simulink model "TimeDelay_DiffParameters"  (R2019b)
settings: Solver=VariableStepAuto  StartTime=0.0  StopTime=1500  RelTol=1e-3
values from neighbouring files (symbols this model uses):
  tau1 = 15    [SmithControl.m]    (also in TimeDelayParameters.m; positivity_matrix.m)
  tau2 = 20    [SmithControl.m]    (also in TimeDelayParameters.m = 30; positivity_matrix.m = 30)
  th1 = 0.85    [AP_TimeDelay.m]    (also in SmithControl.m; TimeDelayParameters.m = 0.32; positivity_matrix.m; rscale.m)
  th2 = 50    [AP_TimeDelay.m]    (also in SmithControl.m; TimeDelayParameters.m; positivity_matrix.m; rscale.m)
  th3 = 60    [AP_TimeDelay.m]    (also in SmithControl.m; TimeDelayParameters.m = 70; positivity_matrix.m; rscale.m)
  th4 = 5    [AP_TimeDelay.m]    (also in SmithControl.m; TimeDelayParameters.m = 2.7; positivity_matrix.m; rscale.m)
  th5 = 20    [AP_TimeDelay.m]    (also in SmithControl.m; TimeDelayParameters.m = 22; positivity_matrix.m; rscale.m)
settings Model: Creator=akshita_jain  LastModifiedBy=akshita_jain

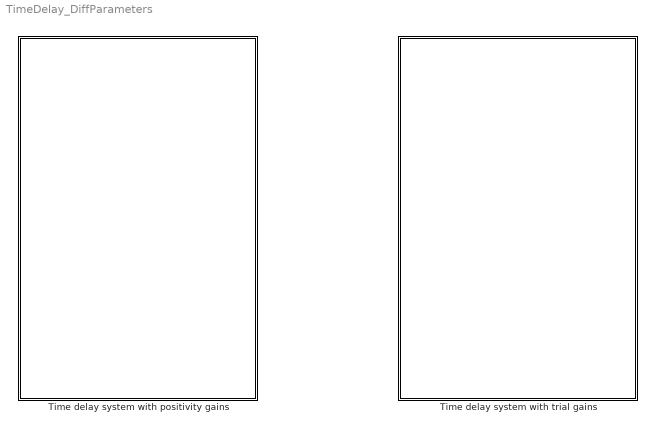
== system TimeDelay_DiffParameters ==
  Time delay system with positivity gains : Subsystem
  Time delay system with trial gains : Subsystem

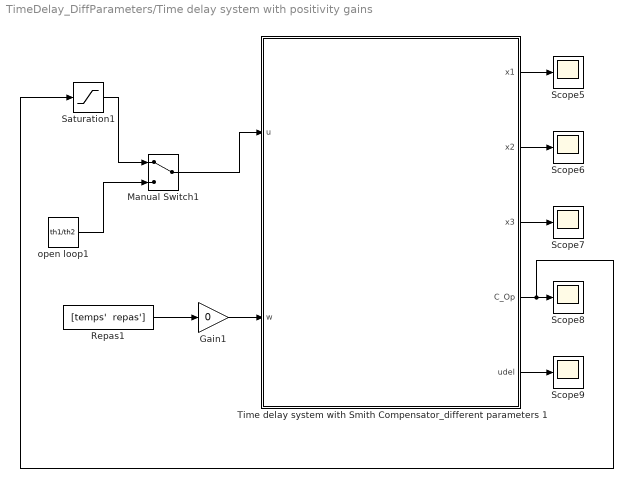
== system TimeDelay_DiffParameters/Time delay system with positivity gains ==
  Gain1 : Gain  Gain=0
  Manual Switch1 : ManualSwitch
  Repas1 : FromWorkspace  VariableName="[temps'  repas']"  SampleTime=0
  Saturation1 : Saturate  UpperLimit=2  LowerLimit=0
  Scope{5..9} (5 alike) : Scope
  Time delay system with Smith Compensator_different parameters 1 : Subsystem
  open loop1 : Constant  Value=th1/th2
  wires:
  Manual Switch1/1 -> Time delay system with Smith Compensator_different parameters 1/1(u)
  Gain1/1 -> Time delay system with Smith Compensator_different parameters 1/2(w)
  Time delay system with Smith Compensator_different parameters 1/3(x3) -> Scope7/1
  Time delay system with Smith Compensator_different parameters 1/2(x2) -> Scope6/1
  Time delay system with Smith Compensator_different parameters 1/5(udel) -> Scope9/1
  Saturation1/1 -> Manual Switch1/1
  Time delay system with Smith Compensator_different parameters 1/1(x1) -> Scope5/1
  Time delay system with Smith Compensator_different parameters 1/4(C_Op) -> Saturation1/1, Scope8/1
  Repas1/1 -> Gain1/1
  open loop1/1 -> Manual Switch1/2

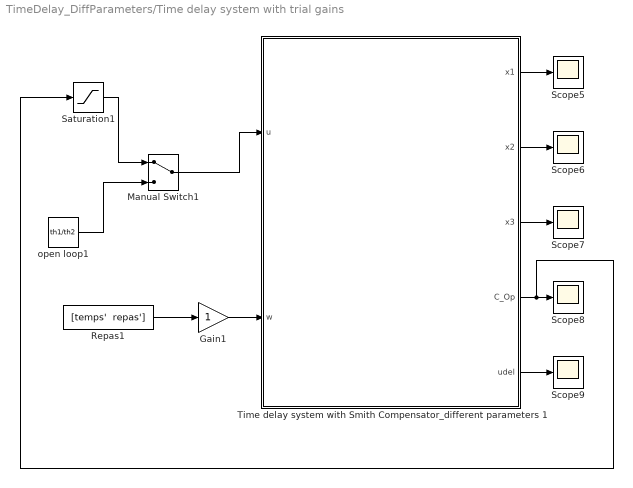
== system TimeDelay_DiffParameters/Time delay system with trial gains ==
  Gain1 : Gain
  Manual Switch1 : ManualSwitch
  Repas1 : FromWorkspace  VariableName="[temps'  repas']"  SampleTime=0
  Saturation1 : Saturate  UpperLimit=2  LowerLimit=0
  Scope{5..9} (5 alike) : Scope
  Time delay system with Smith Compensator_different parameters 1 : Subsystem
  open loop1 : Constant  Value=th1/th2
  wires:
  Manual Switch1/1 -> Time delay system with Smith Compensator_different parameters 1/1(u)
  Gain1/1 -> Time delay system with Smith Compensator_different parameters 1/2(w)
  Time delay system with Smith Compensator_different parameters 1/3(x3) -> Scope7/1
  Time delay system with Smith Compensator_different parameters 1/2(x2) -> Scope6/1
  Time delay system with Smith Compensator_different parameters 1/5(udel) -> Scope9/1
  Saturation1/1 -> Manual Switch1/1
  Time delay system with Smith Compensator_different parameters 1/1(x1) -> Scope5/1
  Time delay system with Smith Compensator_different parameters 1/4(C_Op) -> Saturation1/1, Scope8/1
  Repas1/1 -> Gain1/1
  open loop1/1 -> Manual Switch1/2

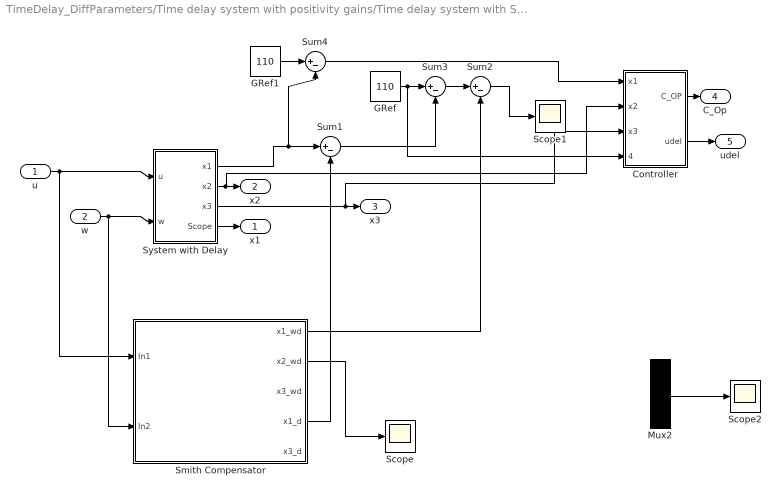
== system TimeDelay_DiffParameters/Time delay system with positivity gains/Time delay system with Smith Compensator_different parameters 1 ==
  u : Inport
  w : Inport  Port=2
  "Controller " : Subsystem
  GRef : Constant  Value=110
  GRef1 : Constant  Value=110
  Mux2 : Mux
  Scope : Scope
  Scope1 : Scope
  Scope2 : Scope
  Smith Compensator : Subsystem
  Sum{1..4} (4 alike) : Sum  Inputs=|+-
  System with Delay : Subsystem
  x1 : Outport
  x2 : Outport  Port=2
  x3 : Outport  Port=3
  C_Op : Outport  Port=4
  udel : Outport  Port=5
  wires:
  u/1 -> Smith Compensator/1(In1), System with Delay/1(u)
  w/1 -> Smith Compensator/2(In2), System with Delay/2(w)
  System with Delay/4(Scope) -> x1/1
  System with Delay/1(x1) -> Sum1/1, Sum4/2
  Smith Compensator/4(x1_d) -> Sum1/2
  Smith Compensator/1(x1_wd) -> Sum2/2
  Sum2/1 -> Scope1/1
  GRef/1 -> "Controller "/4(x1_ref), Sum3/1
  System with Delay/2(x2) -> "Controller "/2(x2), x2/1
  System with Delay/3(x3) -> "Controller "/3(x3), x3/1
  "Controller "/1(C_OP) -> C_Op/1
  "Controller "/2(udel) -> udel/1
  Mux2/1 -> Scope2/1
  Smith Compensator/2(x2_wd) -> Scope/1
  Sum3/1 -> Sum2/1
  GRef1/1 -> Sum4/1
  Sum1/1 -> Sum3/2
  Sum4/1 -> "Controller "/1(x1)

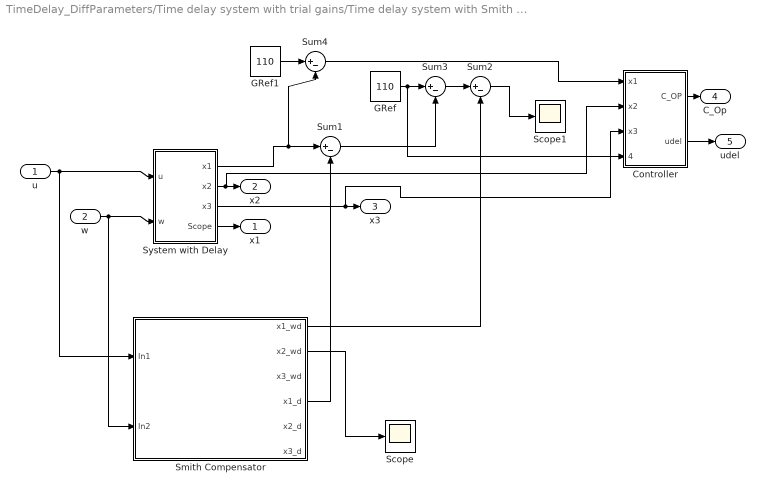
== system TimeDelay_DiffParameters/Time delay system with trial gains/Time delay system with Smith Compensator_different parameters 1 ==
  u : Inport
  w : Inport  Port=2
  "Controller " : Subsystem
  GRef : Constant  Value=110
  GRef1 : Constant  Value=110
  Scope : Scope
  Scope1 : Scope
  Smith Compensator : Subsystem
  Sum{1..4} (4 alike) : Sum  Inputs=|+-
  System with Delay : Subsystem
  x1 : Outport
  x2 : Outport  Port=2
  x3 : Outport  Port=3
  C_Op : Outport  Port=4
  udel : Outport  Port=5
  wires:
  u/1 -> Smith Compensator/1(In1), System with Delay/1(u)
  w/1 -> Smith Compensator/2(In2), System with Delay/2(w)
  System with Delay/4(Scope) -> x1/1
  System with Delay/1(x1) -> Sum1/1, Sum4/2
  Smith Compensator/4(x1_d) -> Sum1/2
  Smith Compensator/1(x1_wd) -> Sum2/2
  Sum2/1 -> Scope1/1
  GRef/1 -> "Controller "/4(x1_ref), Sum3/1
  System with Delay/2(x2) -> "Controller "/2(x2), x2/1
  System with Delay/3(x3) -> "Controller "/3(x3), x3/1
  "Controller "/1(C_OP) -> C_Op/1
  "Controller "/2(udel) -> udel/1
  Smith Compensator/2(x2_wd) -> Scope/1
  Sum3/1 -> Sum2/1
  GRef1/1 -> Sum4/1
  Sum1/1 -> Sum3/2
  Sum4/1 -> "Controller "/1(x1)

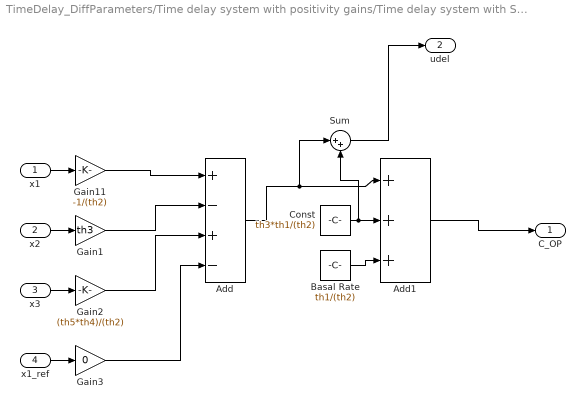
== system TimeDelay_DiffParameters/Time delay system with positivity gains/Time delay system with Smith Compensator_different parameters 1/Controller  ==
  x1 : Inport
  x2 : Inport  Port=2
  x3 : Inport  Port=3
  x1_ref : Inport  Port=4
  Add : Sum  Inputs=+-+-
  Add1 : Sum  Inputs=+++
  Basal Rate : Constant  Value=th1/(th2)  VectorParams1D=off
  Const : Constant  Value=th3*th1/(th2)  VectorParams1D=off
  Gain1 : Gain  Gain=th3
  Gain11 : Gain  Gain=-1/(th2)
  Gain2 : Gain  Gain=(th5*th4)/(th2)
  Gain3 : Gain  Gain=0
  Sum : Sum  Inputs=|++
  C_OP : Outport
  udel : Outport  Port=2
  wires:
  x1/1 -> Gain11/1
  x2/1 -> Gain1/1
  x3/1 -> Gain2/1
  Gain11/1 -> Add/1
  Gain1/1 -> Add/2
  Gain2/1 -> Add/3
  Add/1 -> Sum/1, Add1/1
  Const/1 -> Add1/2, Sum/2
  Basal Rate/1 -> Add1/3
  Add1/1 -> C_OP/1
  Sum/1 -> udel/1
  x1_ref/1 -> Gain3/1
  Gain3/1 -> Add/4

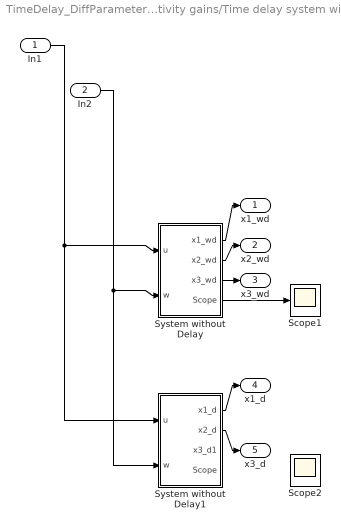
== system TimeDelay_DiffParameters/Time delay system with positivity gains/Time delay system with Smith Compensator_different parameters 1/Smith Compensator ==
  In1 : Inport
  In2 : Inport  Port=2
  Scope1 : Scope
  Scope2 : Scope
  System without Delay : Subsystem
  System without Delay1 : Subsystem
  x1_wd : Outport
  x2_wd : Outport  Port=2
  x3_wd : Outport  Port=3
  x1_d : Outport  Port=4
  x3_d : Outport  Port=5
  wires:
  System without Delay/3(x3_wd) -> x3_wd/1
  System without Delay/2(x2_wd) -> x2_wd/1
  System without Delay/4(Scope) -> Scope1/1
  System without Delay1/1(x1_d) -> x1_d/1
  System without Delay/1(x1_wd) -> x1_wd/1
  System without Delay1/2(x2_d) -> x3_d/1
  In2/1 -> System without Delay1/2(w), System without Delay/2(w)
  In1/1 -> System without Delay1/1(u), System without Delay/1(u)

== system TimeDelay_DiffParameters/Time delay system with positivity gains/Time delay system with Smith Compensator_different parameters 1/System with Delay ==
  u : Inport
  w : Inport  Port=2
  CHO : Subsystem
  Glucose : Subsystem
  Insulin Plasma : Subsystem
  x1 : Outport
  x2 : Outport  Port=2
  x3 : Outport  Port=3
  Scope : Outport  Port=4
  wires:
  Glucose/1(Out1) -> Scope/1
  Glucose/2(x1) -> x1/1
  w/1 -> CHO/1(w)
  Insulin Plasma/1(x2) -> x2/1, Glucose/1(x2)
  u/1 -> Insulin Plasma/1(u)
  CHO/1(x3) -> x3/1, Glucose/2(x3)

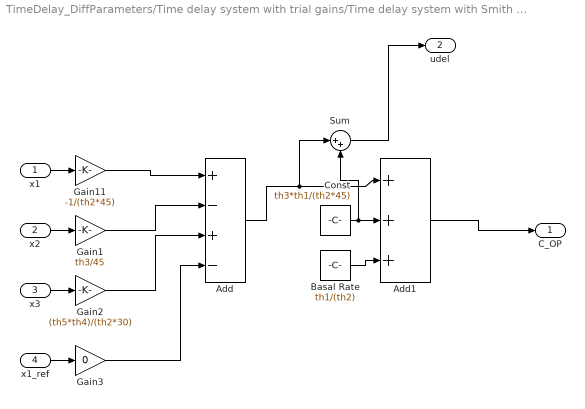
== system TimeDelay_DiffParameters/Time delay system with trial gains/Time delay system with Smith Compensator_different parameters 1/Controller  ==
  x1 : Inport
  x2 : Inport  Port=2
  x3 : Inport  Port=3
  x1_ref : Inport  Port=4
  Add : Sum  Inputs=+-+-
  Add1 : Sum  Inputs=+++
  Basal Rate : Constant  Value=th1/(th2)  VectorParams1D=off
  Const : Constant  Value=th3*th1/(th2*45)  VectorParams1D=off
  Gain1 : Gain  Gain=th3/45
  Gain11 : Gain  Gain=-1/(th2*45)
  Gain2 : Gain  Gain=(th5*th4)/(th2*30)
  Gain3 : Gain  Gain=0
  Sum : Sum  Inputs=|++
  C_OP : Outport
  udel : Outport  Port=2
  wires:
  x1/1 -> Gain11/1
  x2/1 -> Gain1/1
  x3/1 -> Gain2/1
  Gain11/1 -> Add/1
  Gain1/1 -> Add/2
  Gain2/1 -> Add/3
  Add/1 -> Sum/1, Add1/1
  Const/1 -> Add1/2, Sum/2
  Basal Rate/1 -> Add1/3
  Add1/1 -> C_OP/1
  Sum/1 -> udel/1
  x1_ref/1 -> Gain3/1
  Gain3/1 -> Add/4

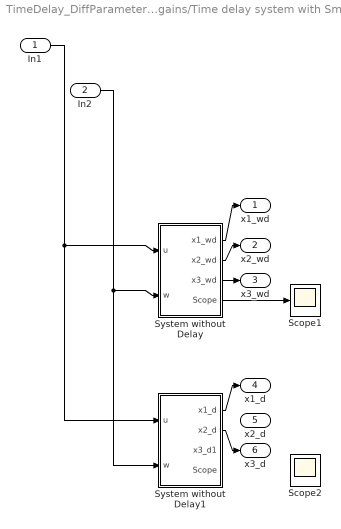
== system TimeDelay_DiffParameters/Time delay system with trial gains/Time delay system with Smith Compensator_different parameters 1/Smith Compensator ==
  In1 : Inport
  In2 : Inport  Port=2
  Scope1 : Scope
  Scope2 : Scope
  System without Delay : Subsystem
  System without Delay1 : Subsystem
  x1_wd : Outport
  x2_wd : Outport  Port=2
  x3_wd : Outport  Port=3
  x1_d : Outport  Port=4
  x2_d : Outport  Port=5
  x3_d : Outport  Port=6
  wires:
  System without Delay/3(x3_wd) -> x3_wd/1
  System without Delay/2(x2_wd) -> x2_wd/1
  System without Delay/4(Scope) -> Scope1/1
  System without Delay1/1(x1_d) -> x1_d/1
  System without Delay/1(x1_wd) -> x1_wd/1
  System without Delay1/2(x2_d) -> x3_d/1
  In2/1 -> System without Delay1/2(w), System without Delay/2(w)
  In1/1 -> System without Delay1/1(u), System without Delay/1(u)

== system TimeDelay_DiffParameters/Time delay system with trial gains/Time delay system with Smith Compensator_different parameters 1/System with Delay ==
  u : Inport
  w : Inport  Port=2
  CHO : Subsystem
  Glucose : Subsystem
  Insulin Plasma : Subsystem
  Scope1 : Scope
  x1 : Outport
  x2 : Outport  Port=2
  x3 : Outport  Port=3
  Scope : Outport  Port=4
  wires:
  Glucose/1(Out1) -> Scope/1
  Glucose/2(x1) -> x1/1
  w/1 -> CHO/1(w)
  Insulin Plasma/1(x2) -> Scope1/1, x2/1, Glucose/1(x2)
  CHO/1(x3) -> x3/1, Glucose/2(x3)
  u/1 -> Insulin Plasma/1(u)

== system TimeDelay_DiffParameters/Time delay system with positivity gains/Time delay system with Smith Compensator_different parameters 1/Smith Compensator/System without Delay ==
  u : Inport
  w : Inport  Port=2
  CHO : Subsystem
  Glucose : Subsystem
  Insulin Plasma : Subsystem
  x1_wd : Outport
  x2_wd : Outport  Port=2
  x3_wd : Outport  Port=3
  Scope : Outport  Port=4
  wires:
  Glucose/2(x1) -> x1_wd/1
  w/1 -> CHO/1(In2)
  Insulin Plasma/1(x2) -> x2_wd/1, Glucose/1(In1)
  u/1 -> Insulin Plasma/1(In1)
  CHO/1(x3) -> x3_wd/1, Glucose/2(In2)
  Glucose/1(Out1) -> Scope/1

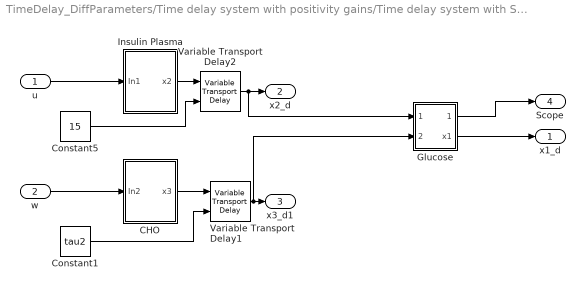
== system TimeDelay_DiffParameters/Time delay system with positivity gains/Time delay system with Smith Compensator_different parameters 1/Smith Compensator/System without Delay1 ==
  u : Inport
  w : Inport  Port=2
  CHO : Subsystem
  Constant1 : Constant  Value=tau2
  Constant5 : Constant  Value=15
  Glucose : Subsystem
  Insulin Plasma : Subsystem
  Variable Transport Delay1 : VariableTransportDelay  VariableDelayType=Variable transport delay  MaximumDelay=30
  Variable Transport Delay2 : VariableTransportDelay  VariableDelayType=Variable transport delay  MaximumDelay=20  InitialOutput=0.0167
  x1_d : Outport
  x2_d : Outport  Port=2
  x3_d1 : Outport  Port=3
  Scope : Outport  Port=4
  wires:
  Glucose/2(x1) -> x1_d/1
  w/1 -> CHO/1(In2)
  u/1 -> Insulin Plasma/1(In1)
  Variable Transport Delay2/1 -> x2_d/1, Glucose/1(In1)
  Insulin Plasma/1(x2) -> Variable Transport Delay2/1
  Constant5/1 -> Variable Transport Delay2/2
  CHO/1(x3) -> Variable Transport Delay1/1
  Variable Transport Delay1/1 -> x3_d1/1, Glucose/2(In2)
  Constant1/1 -> Variable Transport Delay1/2
  Glucose/1(Out1) -> Scope/1

== system TimeDelay_DiffParameters/Time delay system with positivity gains/Time delay system with Smith Compensator_different parameters 1/System with Delay/CHO ==
  w : Inport
  Add6 : Sum  Inputs=-+
  Constant6 : Constant  Value=30  VectorParams1D=off
  Gain12 : Gain  Gain=1/th5
  Gain13 : Gain  Gain=1/th5
  Integrator6 : Integrator  ZeroCross=off
  Variable Transport Delay3 : VariableTransportDelay  VariableDelayType=Variable transport delay  MaximumDelay=30
  x3 : Outport
  wires:
  Variable Transport Delay3/1 -> Gain12/1
  w/1 -> Variable Transport Delay3/1
  Integrator6/1 -> x3/1, Gain13/1
  Add6/1 -> Integrator6/1
  Constant6/1 -> Variable Transport Delay3/2
  Gain13/1 -> Add6/1
  Gain12/1 -> Add6/2

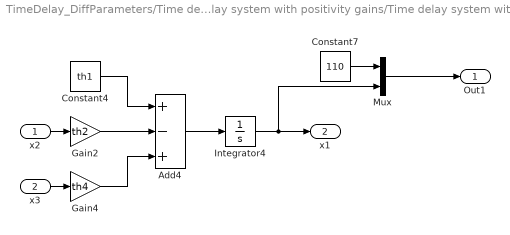
== system TimeDelay_DiffParameters/Time delay system with positivity gains/Time delay system with Smith Compensator_different parameters 1/System with Delay/Glucose ==
  x2 : Inport
  x3 : Inport  Port=2
  Add4 : Sum  Inputs=+-+
  Constant4 : Constant  Value=th1  VectorParams1D=off
  Constant7 : Constant  Value=110  VectorParams1D=off
  Gain2 : Gain  Gain=th2
  Gain4 : Gain  Gain=th4
  Integrator4 : Integrator  InitialCondition=110  ZeroCross=off
  Mux : Mux  Inputs=2
  Out1 : Outport
  x1 : Outport  Port=2
  wires:
  Gain2/1 -> Add4/2
  x3/1 -> Gain4/1
  x2/1 -> Gain2/1
  Mux/1 -> Out1/1
  Add4/1 -> Integrator4/1
  Constant4/1 -> Add4/1
  Integrator4/1 -> x1/1, Mux/2
  Gain4/1 -> Add4/3
  Constant7/1 -> Mux/1

== system TimeDelay_DiffParameters/Time delay system with positivity gains/Time delay system with Smith Compensator_different parameters 1/System with Delay/Insulin Plasma ==
  u : Inport
  Add5 : Sum  Inputs=-+
  Constant5 : Constant  Value=tau1
  Gain10 : Gain  Gain=1/th3
  Gain11 : Gain  Gain=1/th3
  Integrator5 : Integrator  InitialCondition=th1/(th2)  ZeroCross=off
  Variable Transport Delay2 : VariableTransportDelay  VariableDelayType=Variable transport delay  MaximumDelay=20
  x2 : Outport
  wires:
  Add5/1 -> Integrator5/1
  Gain11/1 -> Add5/1
  Gain10/1 -> Add5/2
  Constant5/1 -> Variable Transport Delay2/2
  Integrator5/1 -> x2/1, Gain11/1
  u/1 -> Variable Transport Delay2/1
  Variable Transport Delay2/1 -> Gain10/1

== system TimeDelay_DiffParameters/Time delay system with trial gains/Time delay system with Smith Compensator_different parameters 1/Smith Compensator/System without Delay ==
  u : Inport
  w : Inport  Port=2
  CHO : Subsystem
  Glucose : Subsystem
  Insulin Plasma : Subsystem
  x1_wd : Outport
  x2_wd : Outport  Port=2
  x3_wd : Outport  Port=3
  Scope : Outport  Port=4
  wires:
  Glucose/2(x1) -> x1_wd/1
  w/1 -> CHO/1(In2)
  Insulin Plasma/1(x2) -> x2_wd/1, Glucose/1(In1)
  u/1 -> Insulin Plasma/1(In1)
  CHO/1(x3) -> x3_wd/1, Glucose/2(In2)
  Glucose/1(Out1) -> Scope/1

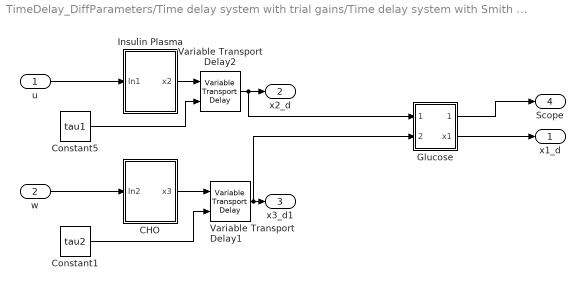
== system TimeDelay_DiffParameters/Time delay system with trial gains/Time delay system with Smith Compensator_different parameters 1/Smith Compensator/System without Delay1 ==
  u : Inport
  w : Inport  Port=2
  CHO : Subsystem
  Constant1 : Constant  Value=tau2
  Constant5 : Constant  Value=tau1
  Glucose : Subsystem
  Insulin Plasma : Subsystem
  Variable Transport Delay1 : VariableTransportDelay  VariableDelayType=Variable transport delay  MaximumDelay=30
  Variable Transport Delay2 : VariableTransportDelay  VariableDelayType=Variable transport delay  MaximumDelay=20
  x1_d : Outport
  x2_d : Outport  Port=2
  x3_d1 : Outport  Port=3
  Scope : Outport  Port=4
  wires:
  Glucose/2(x1) -> x1_d/1
  w/1 -> CHO/1(In2)
  u/1 -> Insulin Plasma/1(In1)
  Variable Transport Delay2/1 -> x2_d/1, Glucose/1(In1)
  Insulin Plasma/1(x2) -> Variable Transport Delay2/1
  Constant5/1 -> Variable Transport Delay2/2
  CHO/1(x3) -> Variable Transport Delay1/1
  Variable Transport Delay1/1 -> x3_d1/1, Glucose/2(In2)
  Constant1/1 -> Variable Transport Delay1/2
  Glucose/1(Out1) -> Scope/1

== system TimeDelay_DiffParameters/Time delay system with trial gains/Time delay system with Smith Compensator_different parameters 1/System with Delay/CHO ==
  w : Inport
  Add6 : Sum  Inputs=-+
  Constant6 : Constant  Value=30  VectorParams1D=off
  Gain12 : Gain  Gain=1/th5
  Gain13 : Gain  Gain=1/th5
  Integrator6 : Integrator  ZeroCross=off
  Variable Transport Delay3 : VariableTransportDelay  VariableDelayType=Variable transport delay  MaximumDelay=30
  x3 : Outport
  wires:
  Variable Transport Delay3/1 -> Gain12/1
  w/1 -> Variable Transport Delay3/1
  Integrator6/1 -> x3/1, Gain13/1
  Add6/1 -> Integrator6/1
  Constant6/1 -> Variable Transport Delay3/2
  Gain13/1 -> Add6/1
  Gain12/1 -> Add6/2

== system TimeDelay_DiffParameters/Time delay system with trial gains/Time delay system with Smith Compensator_different parameters 1/System with Delay/Glucose ==
  x2 : Inport
  x3 : Inport  Port=2
  Add4 : Sum  Inputs=+-+
  Constant4 : Constant  Value=th1  VectorParams1D=off
  Constant7 : Constant  Value=110  VectorParams1D=off
  Gain2 : Gain  Gain=th2
  Gain4 : Gain  Gain=th4
  Integrator4 : Integrator  InitialCondition=110  ZeroCross=off
  Mux : Mux  Inputs=2
  Out1 : Outport
  x1 : Outport  Port=2
  wires:
  Gain2/1 -> Add4/2
  x3/1 -> Gain4/1
  x2/1 -> Gain2/1
  Mux/1 -> Out1/1
  Add4/1 -> Integrator4/1
  Constant4/1 -> Add4/1
  Integrator4/1 -> x1/1, Mux/2
  Gain4/1 -> Add4/3
  Constant7/1 -> Mux/1

== system TimeDelay_DiffParameters/Time delay system with trial gains/Time delay system with Smith Compensator_different parameters 1/System with Delay/Insulin Plasma ==
  u : Inport
  Add5 : Sum  Inputs=-+
  Constant5 : Constant  Value=tau1
  Gain10 : Gain  Gain=th1/th2*th3
  Gain11 : Gain  Gain=1/th3
  Integrator5 : Integrator  InitialCondition=th1/(th2)  ZeroCross=off
  Variable Transport Delay2 : VariableTransportDelay  VariableDelayType=Variable transport delay  MaximumDelay=20  InitialOutput=th1/th2
  x2 : Outport
  wires:
  Gain11/1 -> Add5/1
  Gain10/1 -> Add5/2
  Constant5/1 -> Variable Transport Delay2/2
  u/1 -> Variable Transport Delay2/1
  Variable Transport Delay2/1 -> Gain10/1
  Integrator5/1 -> x2/1, Gain11/1
  Add5/1 -> Integrator5/1

== system TimeDelay_DiffParameters/Time delay system with positivity gains/Time delay system with Smith Compensator_different parameters 1/Smith Compensator/System without Delay/CHO ==
  In2 : Inport
  Add6 : Sum  Inputs=-+
  Gain12 : Gain  Gain=1/th5
  Gain13 : Gain  Gain=1/th5
  Integrator6 : Integrator  ZeroCross=off
  x3 : Outport
  wires:
  In2/1 -> Gain12/1
  Integrator6/1 -> x3/1, Gain13/1
  Add6/1 -> Integrator6/1
  Gain13/1 -> Add6/1
  Gain12/1 -> Add6/2

== system TimeDelay_DiffParameters/Time delay system with positivity gains/Time delay system with Smith Compensator_different parameters 1/Smith Compensator/System without Delay/Glucose ==
  In1 : Inport
  In2 : Inport  Port=2
  Add4 : Sum  Inputs=+-+
  Constant4 : Constant  Value=th1  VectorParams1D=off
  Constant7 : Constant  Value=110  VectorParams1D=off
  Gain2 : Gain  Gain=th2
  Gain4 : Gain  Gain=th4
  Integrator4 : Integrator  InitialCondition=110  ZeroCross=off
  Mux : Mux  Inputs=2
  Out1 : Outport
  x1 : Outport  Port=2
  wires:
  Gain2/1 -> Add4/2
  In2/1 -> Gain4/1
  In1/1 -> Gain2/1
  Mux/1 -> Out1/1
  Add4/1 -> Integrator4/1
  Constant4/1 -> Add4/1
  Integrator4/1 -> x1/1, Mux/2
  Gain4/1 -> Add4/3
  Constant7/1 -> Mux/1

== system TimeDelay_DiffParameters/Time delay system with positivity gains/Time delay system with Smith Compensator_different parameters 1/Smith Compensator/System without Delay/Insulin Plasma ==
  In1 : Inport
  Add5 : Sum  Inputs=-+
  Gain10 : Gain  Gain=1/th3
  Gain11 : Gain  Gain=1/th3
  Integrator5 : Integrator  InitialCondition=0.017  ZeroCross=off
  x2 : Outport
  wires:
  Add5/1 -> Integrator5/1
  Gain11/1 -> Add5/1
  In1/1 -> Gain10/1
  Gain10/1 -> Add5/2
  Integrator5/1 -> x2/1, Gain11/1

== system TimeDelay_DiffParameters/Time delay system with positivity gains/Time delay system with Smith Compensator_different parameters 1/Smith Compensator/System without Delay1/CHO ==
  In2 : Inport
  Add6 : Sum  Inputs=-+
  Gain12 : Gain  Gain=1/th5
  Gain13 : Gain  Gain=1/th5
  Integrator6 : Integrator  ZeroCross=off
  x3 : Outport
  wires:
  In2/1 -> Gain12/1
  Integrator6/1 -> x3/1, Gain13/1
  Add6/1 -> Integrator6/1
  Gain13/1 -> Add6/1
  Gain12/1 -> Add6/2

== system TimeDelay_DiffParameters/Time delay system with positivity gains/Time delay system with Smith Compensator_different parameters 1/Smith Compensator/System without Delay1/Glucose ==
  In1 : Inport
  In2 : Inport  Port=2
  Add4 : Sum  Inputs=+-+
  Constant4 : Constant  Value=th1  VectorParams1D=off
  Constant7 : Constant  Value=110  VectorParams1D=off
  Gain2 : Gain  Gain=th2
  Gain4 : Gain  Gain=th4
  Integrator4 : Integrator  InitialCondition=110  ZeroCross=off
  Mux : Mux  Inputs=2
  Out1 : Outport
  x1 : Outport  Port=2
  wires:
  Gain2/1 -> Add4/2
  In2/1 -> Gain4/1
  In1/1 -> Gain2/1
  Mux/1 -> Out1/1
  Add4/1 -> Integrator4/1
  Constant4/1 -> Add4/1
  Integrator4/1 -> x1/1, Mux/2
  Gain4/1 -> Add4/3
  Constant7/1 -> Mux/1

== system TimeDelay_DiffParameters/Time delay system with positivity gains/Time delay system with Smith Compensator_different parameters 1/Smith Compensator/System without Delay1/Insulin Plasma ==
  In1 : Inport
  Add5 : Sum  Inputs=-+
  Gain10 : Gain  Gain=1/th3
  Gain11 : Gain  Gain=1/th3
  Integrator5 : Integrator  InitialCondition=0.017  ZeroCross=off
  x2 : Outport
  wires:
  Add5/1 -> Integrator5/1
  Gain11/1 -> Add5/1
  In1/1 -> Gain10/1
  Gain10/1 -> Add5/2
  Integrator5/1 -> x2/1, Gain11/1

== system TimeDelay_DiffParameters/Time delay system with trial gains/Time delay system with Smith Compensator_different parameters 1/Smith Compensator/System without Delay/CHO ==
  In2 : Inport
  Add6 : Sum  Inputs=-+
  Gain12 : Gain  Gain=1/th5
  Gain13 : Gain  Gain=1/th5
  Integrator6 : Integrator  ZeroCross=off
  x3 : Outport
  wires:
  In2/1 -> Gain12/1
  Integrator6/1 -> x3/1, Gain13/1
  Add6/1 -> Integrator6/1
  Gain13/1 -> Add6/1
  Gain12/1 -> Add6/2

== system TimeDelay_DiffParameters/Time delay system with trial gains/Time delay system with Smith Compensator_different parameters 1/Smith Compensator/System without Delay/Glucose ==
  In1 : Inport
  In2 : Inport  Port=2
  Add4 : Sum  Inputs=+-+
  Constant4 : Constant  Value=th1  VectorParams1D=off
  Constant7 : Constant  Value=110  VectorParams1D=off
  Gain2 : Gain  Gain=th2
  Gain4 : Gain  Gain=th4
  Integrator4 : Integrator  InitialCondition=110  ZeroCross=off
  Mux : Mux  Inputs=2
  Out1 : Outport
  x1 : Outport  Port=2
  wires:
  Gain2/1 -> Add4/2
  In2/1 -> Gain4/1
  In1/1 -> Gain2/1
  Mux/1 -> Out1/1
  Add4/1 -> Integrator4/1
  Constant4/1 -> Add4/1
  Integrator4/1 -> x1/1, Mux/2
  Gain4/1 -> Add4/3
  Constant7/1 -> Mux/1

== system TimeDelay_DiffParameters/Time delay system with trial gains/Time delay system with Smith Compensator_different parameters 1/Smith Compensator/System without Delay/Insulin Plasma ==
  In1 : Inport
  Add5 : Sum  Inputs=-+
  Gain10 : Gain  Gain=1/th3
  Gain11 : Gain  Gain=1/th3
  Integrator5 : Integrator  InitialCondition=0.017  ZeroCross=off
  x2 : Outport
  wires:
  Add5/1 -> Integrator5/1
  Gain11/1 -> Add5/1
  In1/1 -> Gain10/1
  Gain10/1 -> Add5/2
  Integrator5/1 -> x2/1, Gain11/1

== system TimeDelay_DiffParameters/Time delay system with trial gains/Time delay system with Smith Compensator_different parameters 1/Smith Compensator/System without Delay1/CHO ==
  In2 : Inport
  Add6 : Sum  Inputs=-+
  Gain12 : Gain  Gain=1/th5
  Gain13 : Gain  Gain=1/th5
  Integrator6 : Integrator  ZeroCross=off
  x3 : Outport
  wires:
  In2/1 -> Gain12/1
  Integrator6/1 -> x3/1, Gain13/1
  Add6/1 -> Integrator6/1
  Gain13/1 -> Add6/1
  Gain12/1 -> Add6/2

== system TimeDelay_DiffParameters/Time delay system with trial gains/Time delay system with Smith Compensator_different parameters 1/Smith Compensator/System without Delay1/Glucose ==
  In1 : Inport
  In2 : Inport  Port=2
  Add4 : Sum  Inputs=+-+
  Constant4 : Constant  Value=th1  VectorParams1D=off
  Constant7 : Constant  Value=110  VectorParams1D=off
  Gain2 : Gain  Gain=th2
  Gain4 : Gain  Gain=th4
  Integrator4 : Integrator  InitialCondition=110  ZeroCross=off
  Mux : Mux  Inputs=2
  Out1 : Outport
  x1 : Outport  Port=2
  wires:
  Gain2/1 -> Add4/2
  In2/1 -> Gain4/1
  In1/1 -> Gain2/1
  Mux/1 -> Out1/1
  Add4/1 -> Integrator4/1
  Constant4/1 -> Add4/1
  Integrator4/1 -> x1/1, Mux/2
  Gain4/1 -> Add4/3
  Constant7/1 -> Mux/1

== system TimeDelay_DiffParameters/Time delay system with trial gains/Time delay system with Smith Compensator_different parameters 1/Smith Compensator/System without Delay1/Insulin Plasma ==
  In1 : Inport
  Add5 : Sum  Inputs=-+
  Gain10 : Gain  Gain=1/th3
  Gain11 : Gain  Gain=1/th3
  Integrator5 : Integrator  InitialCondition=0.017  ZeroCross=off
  x2 : Outport
  wires:
  Add5/1 -> Integrator5/1
  Gain11/1 -> Add5/1
  In1/1 -> Gain10/1
  Gain10/1 -> Add5/2
  Integrator5/1 -> x2/1, Gain11/1
